simulink model "s03_PID_emulation_be_ffs"  (R2022b)
settings: Solver=FixedStepAuto  StartTime=0.0  StopTime=10  FixedStep=0.001  RelTol=1e-3
undefined symbols (not defined in the file or in its folder): degs2rpm, der, DiscIntNeverNeededParam, drv, gbox, mot, National_Instruments, PCI, pidz, real, rpm2degs, rpm2rads, sens, simul, T, Ts
libraries: sldrtlib x3, simulink x1
settings Model: SimulationMode=external  ExtModeTrigDuration=1000001  ExtModeTrigDurationFloating=50001  Creator=perondavid  LastModifiedBy=perondavid
settings DataIOCC: LoggingToFile=on
settings HardwareCC: ProdBitPerLong=64  ProdHWDeviceType=Intel->x86-64 (Linux 64)
settings RTWCC: Description=Simulink Desktop Real-Time  SystemTargetFile=sldrt.tlc  TemplateMakefile=sldrt.tmf  RTWCompilerOptimization=on
settings CodeAppCC: MaxIdLength=95
settings SimulinkDesktopRealTimeCC: TargetLibSuffix=_sldrt.a  TargetPreCompLibLocation=C:\Program Files\MATLAB\R2022b\toolbox\sldrt\lib\win64

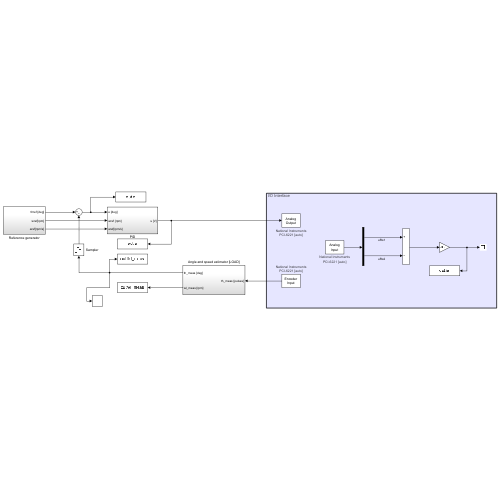
[thumbnail: Simulink's stored preview of the top-level diagram]
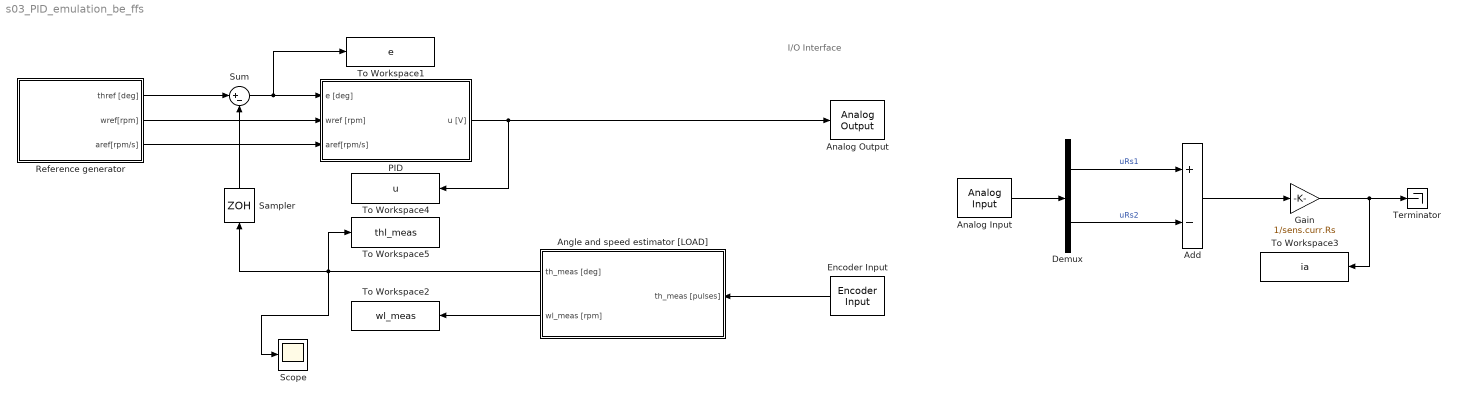
== system s03_PID_emulation_be_ffs ==
  note: I/O Interface
  Add : Sum  Inputs=+-
  Analog Input : sldrtlib/Analog Input  SampleTime=-1  MaxMissedTicks=10  ShowMissedTicks=off  YieldWhenWaiting=off  DrvName=National_Instruments/PCI-6221  DrvAddress=4294967295  DrvOptions=[0 0 0 2 0]  Channels=[1, 2]  RangeMode=1  VoltRange=1  DataType=1
      settings: AttributesFormatString=National Instruments\nPCI-6221 [auto]
  Analog Output : sldrtlib/Analog Output  SampleTime=-1  MaxMissedTicks=10  ShowMissedTicks=off  YieldWhenWaiting=off  DrvName=National_Instruments/PCI-6221  DrvAddress=4294967295  DrvOptions=[0 0 0 2 0]  Channels=1  RangeMode=1  VoltRange=1  InitialValue=0  FinalValue=0
      settings: AttributesFormatString=National Instruments\nPCI-6221 [auto]
  Angle and speed estimator [LOAD] : Subsystem
  Demux : Demux  Outputs=2
  Encoder Input : sldrtlib/Encoder Input  SampleTime=-1  MaxMissedTicks=10  ShowMissedTicks=off  YieldWhenWaiting=off  DrvName=National_Instruments/PCI-6221  DrvAddress=4294967295  DrvOptions=[0 0 0 2 0]  Channels=1  QuadMode=3  IndexPulse=1  InputFilter=Inf  DataType=1
      settings: AttributesFormatString=National Instruments\nPCI-6221 [auto]
  Gain : Gain  Gain=1/sens.curr.Rs
  PID : Subsystem
  Reference generator : Subsystem
  Sampler : ZeroOrderHold  SampleTime=T(simul.Ts_selector)
  Scope : Scope
  Sum : Sum  Inputs=|+-
  Terminator : Terminator
  To Workspace1 : ToWorkspace  VariableName=e  SaveFormat=Structure With Time  SampleTime=Ts
  To Workspace2 : ToWorkspace  VariableName=wl_meas  SaveFormat=Structure With Time  SampleTime=Ts
  To Workspace3 : ToWorkspace  VariableName=ia  SaveFormat=Structure With Time  SampleTime=Ts
  To Workspace4 : ToWorkspace  VariableName=u  SaveFormat=Structure With Time  SampleTime=Ts
  To Workspace5 : ToWorkspace  VariableName=thl_meas  SaveFormat=Structure With Time  SampleTime=Ts
  wires:
  Demux/1 -> Add/1  "uRs1"
  Demux/2 -> Add/2  "uRs2"
  Add/1 -> Gain/1
  Gain/1 -> To Workspace3/1, Terminator/1
  Analog Input/1 -> Demux/1
  Reference generator/2(wref[rpm]) -> PID/2(wref [rpm])
  Angle and speed estimator [LOAD]/2(wl_meas [rpm]) -> To Workspace2/1
  Reference generator/1(thref [deg]) -> Sum/1
  Sampler/1 -> Sum/2
  Reference generator/3(aref[rpm/s]) -> PID/3(aref[rpm/s])
  Sum/1 -> To Workspace1/1, PID/1(e [deg])
  Angle and speed estimator [LOAD]/1(th_meas [deg]) -> Scope/1, Sampler/1, To Workspace5/1
  PID/1(u [V]) -> Analog Output/1, To Workspace4/1
  Encoder Input/1 -> Angle and speed estimator [LOAD]/1(th_meas [pulses])

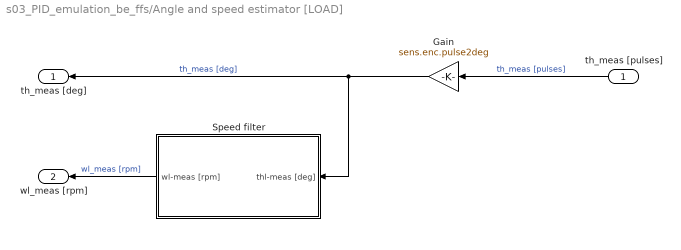
== system s03_PID_emulation_be_ffs/Angle and speed estimator [LOAD] ==
  th_meas [pulses] : Inport
  Gain : Gain  Gain=sens.enc.pulse2deg
  Speed filter : Subsystem
  th_meas [deg] : Outport
  wl_meas [rpm] : Outport  Port=2
  wires:
  Speed filter/1(wl-meas [rpm]) -> wl_meas [rpm]/1  "wl_meas [rpm]"
  th_meas [pulses]/1 -> Gain/1  "th_meas [pulses]"
  Gain/1 -> Speed filter/1(thl-meas [deg]), th_meas [deg]/1  "th_meas [deg]"

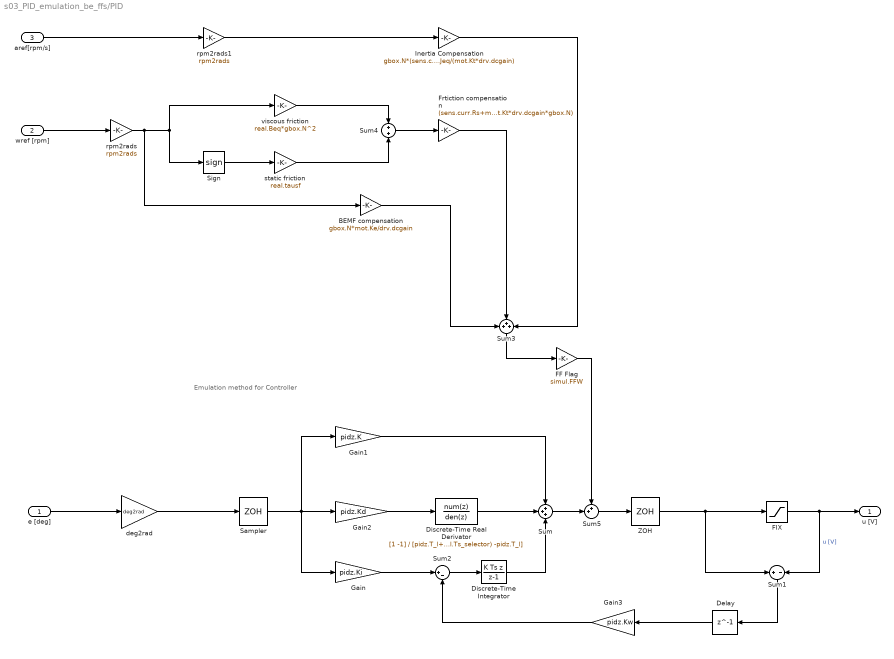
== system s03_PID_emulation_be_ffs/PID ==
  note: Emulation method for Controller
  e [deg] : Inport
  wref [rpm] : Inport  Port=2
  aref[rpm/s] : Inport  Port=3
  BEMF compensation : Gain  Gain=gbox.N*mot.Ke/drv.dcgain
  Delay : Delay  DelayLength=1
  Discrete-Time Integrator : DiscreteIntegrator  IntegratorMethod=Integration: Backward Euler  SampleTime=T(simul.Ts_selector)  ICPrevOutput=DiscIntNeverNeededParam  ICPrevScaledInput=DiscIntNeverNeededParam
  "Discrete-Time Real Derivator " : DiscreteTransferFcn  Numerator=[1 -1]  Denominator=[pidz.T_l+T(simul.Ts_selector) -pidz.T_l]  SampleTime=T(simul.Ts_selector)
  FF Flag : Gain  Gain=simul.FFW
  "FIX " : Saturate  UpperLimit=10  LowerLimit=-10
  Frtiction compensation : Gain  Gain=(sens.curr.Rs+mot.R)/(mot.Kt*drv.dcgain*gbox.N)
  Gain : Gain  Gain=pidz.Ki
  Gain1 : Gain  Gain=pidz.K
  Gain2 : Gain  Gain=pidz.Kd
  Gain3 : Gain  Gain=pidz.Kw
  Inertia Compensation : Gain  Gain=gbox.N*(sens.curr.Rs+mot.R)*real.Jeq/(mot.Kt*drv.dcgain)
  Sampler : ZeroOrderHold  SampleTime=T(simul.Ts_selector)
  Sign : Signum
  Sum : Sum  Inputs=+++
  Sum1 : Sum  Inputs=+|-
  Sum2 : Sum  Inputs=|+-
  Sum3 : Sum  Inputs=+++
  Sum4 : Sum
  Sum5 : Sum  Inputs=++|
  ZOH : ZeroOrderHold  SampleTime=T(simul.Ts_selector)
  deg2rad : Gain  Gain=deg2rad
  rpm2rads : Gain  Gain=rpm2rads
  rpm2rads1 : Gain  Gain=rpm2rads
  static friction : Gain  Gain=real.tausf
  viscous friction : Gain  Gain=real.Beq*gbox.N^2
  u [V] : Outport
  wires:
  e [deg]/1 -> deg2rad/1
  "FIX "/1 -> Sum1/2, u [V]/1  "u [V]"
  deg2rad/1 -> Sampler/1
  ZOH/1 -> Sum1/1, "FIX "/1
  Gain2/1 -> "Discrete-Time Real Derivator "/1
  Sampler/1 -> Gain2/1, Gain1/1, Gain/1
  Gain1/1 -> Sum/1
  "Discrete-Time Real Derivator "/1 -> Sum/2
  Discrete-Time Integrator/1 -> Sum/3
  Gain/1 -> Sum2/1
  Sum2/1 -> Discrete-Time Integrator/1
  Sum1/1 -> Delay/1
  Gain3/1 -> Sum2/2
  static friction/1 -> Sum4/2
  wref [rpm]/1 -> rpm2rads/1
  Sign/1 -> static friction/1
  rpm2rads1/1 -> Inertia Compensation/1
  Inertia Compensation/1 -> Sum3/3
  BEMF compensation/1 -> Sum3/1
  rpm2rads/1 -> BEMF compensation/1, Sign/1, viscous friction/1
  aref[rpm/s]/1 -> rpm2rads1/1
  viscous friction/1 -> Sum4/1
  Frtiction compensation/1 -> Sum3/2
  Sum4/1 -> Frtiction compensation/1
  Sum3/1 -> FF Flag/1
  Sum/1 -> Sum5/2
  FF Flag/1 -> Sum5/1
  Sum5/1 -> ZOH/1
  Delay/1 -> Gain3/1

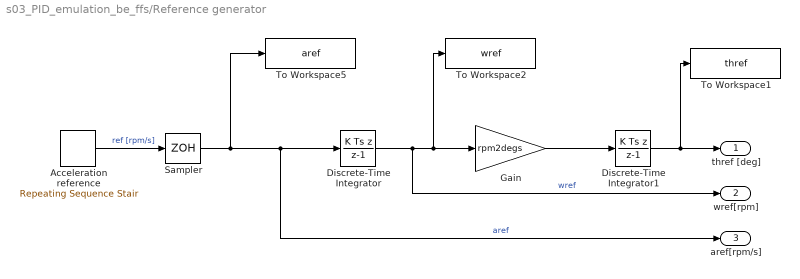
== system s03_PID_emulation_be_ffs/Reference generator ==
  Acceleration reference : simulink/Sources/Repeating Sequence Stair  OutValues=[900 0 -900 -900 0 900].'  tsamp=0.5  OutMin=[]  OutMax=[]  OutDataTypeStr=double  OutputDataTypeScalingMode=double  OutDataType=fixdt(0,8)  ConRadixGroup=Best Precision: Vector-wise  OutScaling=2^-12
  Discrete-Time Integrator : DiscreteIntegrator  IntegratorMethod=Integration: Backward Euler  SampleTime=-1  ICPrevOutput=DiscIntNeverNeededParam  ICPrevScaledInput=DiscIntNeverNeededParam
  Discrete-Time Integrator1 : DiscreteIntegrator  IntegratorMethod=Integration: Backward Euler  SampleTime=-1  ICPrevOutput=DiscIntNeverNeededParam  ICPrevScaledInput=DiscIntNeverNeededParam
  Gain : Gain  Gain=rpm2degs
  Sampler : ZeroOrderHold  SampleTime=T(simul.Ts_selector)
  To Workspace1 : ToWorkspace  VariableName=thref  SaveFormat=Structure With Time  SampleTime=Ts
  To Workspace2 : ToWorkspace  VariableName=wref  SaveFormat=Structure With Time  SampleTime=Ts
  To Workspace5 : ToWorkspace  VariableName=aref  SaveFormat=Structure With Time  SampleTime=Ts
  thref [deg] : Outport
  wref[rpm] : Outport  Port=2
  aref[rpm/s] : Outport  Port=3
  wires:
  Acceleration reference/1 -> Sampler/1  "ref [rpm/s]"
  Sampler/1 -> To Workspace5/1, aref[rpm/s]/1, Discrete-Time Integrator/1  "aref"
  Discrete-Time Integrator/1 -> wref[rpm]/1, To Workspace2/1, Gain/1  "wref"
  Discrete-Time Integrator1/1 -> To Workspace1/1, thref [deg]/1
  Gain/1 -> Discrete-Time Integrator1/1

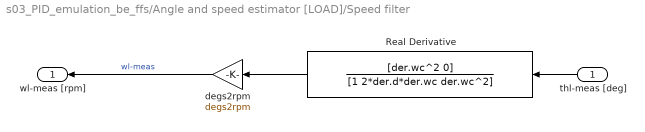
== system s03_PID_emulation_be_ffs/Angle and speed estimator [LOAD]/Speed filter ==
  thl-meas [deg] : Inport
  Real Derivative : TransferFcn  Numerator=[der.wc^2 0]  Denominator=[1 2*der.d*der.wc der.wc^2]
  degs2rpm : Gain  Gain=degs2rpm
  wl-meas [rpm] : Outport
  wires:
  thl-meas [deg]/1 -> Real Derivative/1
  degs2rpm/1 -> wl-meas [rpm]/1  "wl-meas"
  Real Derivative/1 -> degs2rpm/1
